simulink model "Gerador_de_dados_5_1"  (R2013a)
settings: Solver=FixedStepDiscrete  StartTime=0.0  StopTime=800  RelTol=1e-3
values from neighbouring files (symbols this model uses):
  T = 1    [Variaveis.mat]
undefined symbols (not defined in the file or in its folder): St
settings Model: Creator=Élio  LastModifiedBy=Élio
settings OptimizationCC: InlineParams=on

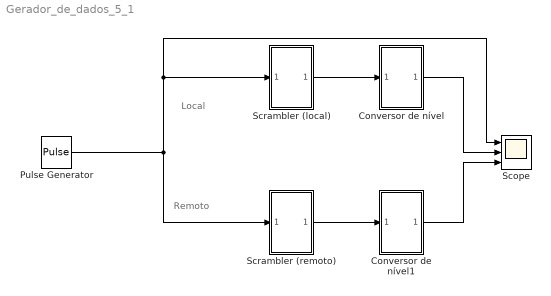
== system Gerador_de_dados_5_1 ==
  note: Remoto
  note: Local
  Conversor de nível : Subsystem
  Conversor de nível1 : Subsystem
  Pulse Generator : DiscretePulseGenerator  PulseType=Time based  Period=2*T  PulseWidth=50  SampleTime=St
  Scope : Scope  NumInputPorts=3
      settings: YMin=-5~-5~-5  YMax=5~5~5
  Scrambler (local) : Subsystem
  Scrambler (remoto) : Subsystem
  wires:
  Pulse Generator/1 -> Scope/1, Scrambler (local)/1(In1), Scrambler (remoto)/1(In1)
  Scrambler (local)/1(Out1) -> Conversor de nível/1(In2)
  Scrambler (remoto)/1(Out1) -> Conversor de nível1/1(In2)
  Conversor de nível1/1(Out2) -> Scope/3
  Conversor de nível/1(Out2) -> Scope/2

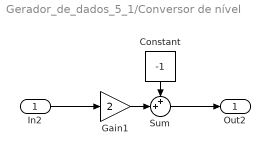
== system Gerador_de_dados_5_1/Conversor de nível ==
  In2 : Inport
  Constant : Constant  Value=-1
  Gain1 : Gain  Gain=2
  Sum : Sum  Inputs=++|
  Out2 : Outport
  wires:
  In2/1 -> Gain1/1
  Sum/1 -> Out2/1
  Gain1/1 -> Sum/2
  Constant/1 -> Sum/1

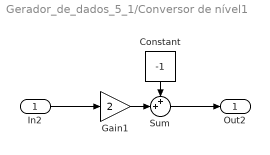
== system Gerador_de_dados_5_1/Conversor de nível1 ==
  In2 : Inport
  Constant : Constant  Value=-1
  Gain1 : Gain  Gain=2
  Sum : Sum  Inputs=++|
  Out2 : Outport
  wires:
  In2/1 -> Gain1/1
  Sum/1 -> Out2/1
  Gain1/1 -> Sum/2
  Constant/1 -> Sum/1

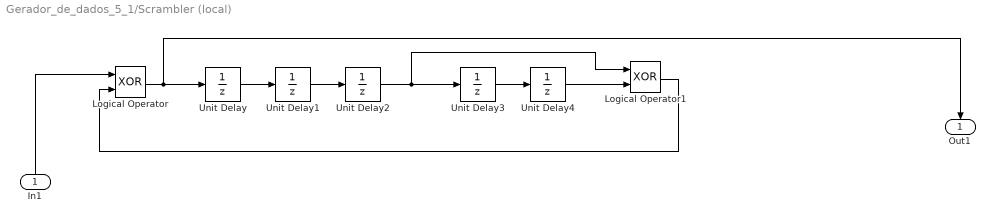
== system Gerador_de_dados_5_1/Scrambler (local) ==
  In1 : Inport
  Logical Operator : Logic  Operator=XOR  AllPortsSameDT=off  OutDataTypeStr=fixdt(1,16)
  Logical Operator1 : Logic  Operator=XOR  AllPortsSameDT=off  OutDataTypeStr=boolean
  Unit Delay{,1..4} (5 alike) : UnitDelay  SampleTime=-1
  Out1 : Outport
  wires:
  In1/1 -> Logical Operator/1
  Logical Operator/1 -> Out1/1, Unit Delay/1
  Unit Delay/1 -> Unit Delay1/1
  Logical Operator1/1 -> Logical Operator/2
  Unit Delay3/1 -> Unit Delay4/1
  Unit Delay4/1 -> Logical Operator1/2
  Unit Delay1/1 -> Unit Delay2/1
  Unit Delay2/1 -> Logical Operator1/1, Unit Delay3/1

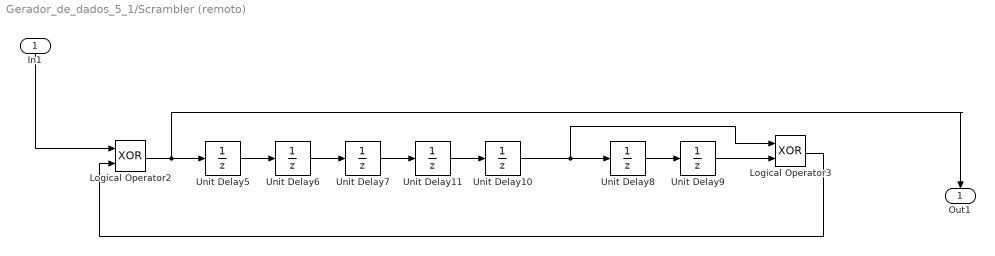
== system Gerador_de_dados_5_1/Scrambler (remoto) ==
  In1 : Inport
  Logical Operator2 : Logic  Operator=XOR  AllPortsSameDT=off  OutDataTypeStr=fixdt(1,16)
  Logical Operator3 : Logic  Operator=XOR  AllPortsSameDT=off  OutDataTypeStr=boolean
  Unit Delay{5..11} (7 alike) : UnitDelay  SampleTime=-1
  Out1 : Outport
  wires:
  In1/1 -> Logical Operator2/1
  Unit Delay6/1 -> Unit Delay7/1
  Unit Delay9/1 -> Logical Operator3/2
  Unit Delay11/1 -> Unit Delay10/1
  Unit Delay10/1 -> Logical Operator3/1, Unit Delay8/1
  Logical Operator3/1 -> Logical Operator2/2
  Unit Delay7/1 -> Unit Delay11/1
  Unit Delay8/1 -> Unit Delay9/1
  Logical Operator2/1 -> Out1/1, Unit Delay5/1
  Unit Delay5/1 -> Unit Delay6/1
